simulink model "SF033A_VehSigCdng"  (R2013b)
settings: Solver=FixedStepDiscrete  StartTime=0.0  StopTime=6  FixedStep=.002  RelTol=1e-3
model workspace (MAT data in the model file):
  SLAMConfig_1_ATPP = [3707764736; 2; 1; 1; 1; 34]
values from neighbouring files (symbols this model uses):
  ARCHGLBPRM_180OVERPI_ULS_F32 = DataDict.Constant    [SF033A_VehSigCdng_DataDict.m]
  ARCHGLBPRM_2MILLISEC_SEC_F32 = DataDict.Constant    [SF033A_VehSigCdng_DataDict.m]
  AUNITCNVN_KPHPERSECPERMTRPERSECSQD_F32 = DataDict.Constant    [SF033A_VehSigCdng_DataDict.m]
  FLTINJ_VEHSIGCDNG_SERLCOMVEHLATA = DataDict.Constant    [SF033A_VehSigCdng_DataDict.m]
  FLTINJ_VEHSIGCDNG_SERLCOMVEHLGTA = DataDict.Constant    [SF033A_VehSigCdng_DataDict.m]
  FLTINJ_VEHSIGCDNG_SERLCOMVEHSPD = DataDict.Constant    [SF033A_VehSigCdng_DataDict.m]
  FLTINJ_VEHSIGCDNG_SERLCOMVEHYAWRATE = DataDict.Constant    [SF033A_VehSigCdng_DataDict.m]
  KPHCONVTOMTRPERSEC_MTRPERSECPERKPH_F32 = DataDict.Constant    [SF033A_VehSigCdng_DataDict.m]
  VehSigCdngDftLatA = DataDict.Calibration    [SF033A_VehSigCdng_DataDict.m]
  VehSigCdngDftLgtA = DataDict.Calibration    [SF033A_VehSigCdng_DataDict.m]
  VehSigCdngDftVehSpd = DataDict.Calibration    [SF033A_VehSigCdng_DataDict.m]
  VehSigCdngDftYawRate = DataDict.Calibration    [SF033A_VehSigCdng_DataDict.m]
  VehSigCdngLatADifThd = DataDict.Calibration    [SF033A_VehSigCdng_DataDict.m]
  VehSigCdngLatASlewRate = DataDict.Calibration    [SF033A_VehSigCdng_DataDict.m]
  VehSigCdngLtgADifThd = DataDict.Calibration    [SF033A_VehSigCdng_DataDict.m]
  VehSigCdngLtgASlewRate = DataDict.Calibration    [SF033A_VehSigCdng_DataDict.m]
  VehSigCdngVehSpdDifThd = DataDict.Calibration    [SF033A_VehSigCdng_DataDict.m]
  VehSigCdngVehSpdSlewRate = DataDict.Calibration    [SF033A_VehSigCdng_DataDict.m]
  VehSigCdngVehYawSlewRate = DataDict.Calibration    [SF033A_VehSigCdng_DataDict.m]
  VehSigCdngYawRateDifThd = DataDict.Calibration    [SF033A_VehSigCdng_DataDict.m]
  VEHSPDOVRDHWTQTHD_HWNWTMTR_F32 = DataDict.Constant    [SF033A_VehSigCdng_DataDict.m]
libraries: NxtrLim x9, Fil x4, simulink x1
(part 2 of 3)

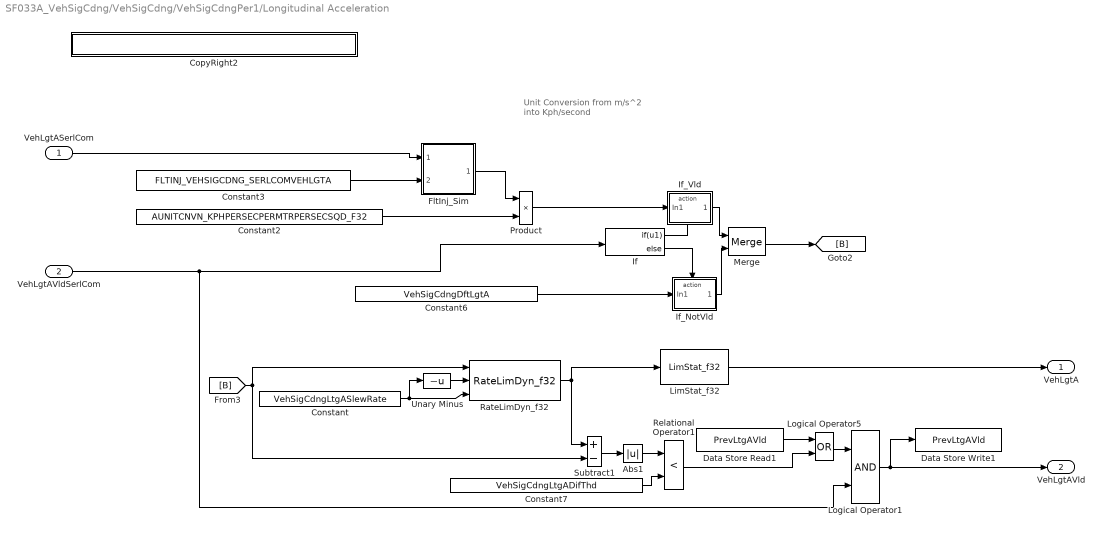
== system SF033A_VehSigCdng/VehSigCdng/VehSigCdngPer1/Longitudinal Acceleration ==
  note: Unit Conversion from
      | m/s^2 into Kph/second
  VehLgtASerlCom : Inport  RequirementInfo="{'linktype_rmi_doors' '00012fc2 (/E-STEER Core/SubSystem Specifications/Application Functions - EA4/SF033A Vehicle Signal Conditioning)' '#SF033A_86' 'true' 'REQ:  SF033A_86' '' ; 'linktype_rmi_doors' '00012fc2 (/E-STEER Core/SubSystem Specifications/Application Functions - EA4/SF033A Vehicle Signal Conditioning)' '#SF033A_82' 'true' 'REQ:  SF033A_82' '' } %GIDa_33bbc02e_3c9f_42eb_b3cb_1f1096c685a4"  PortDimensions=1
  VehLgtAVldSerlCom : Inport  RequirementInfo="{'linktype_rmi_doors' '00012fc2 (/E-STEER Core/SubSystem Specifications/Application Functions - EA4/SF033A Vehicle Signal Conditioning)' '#SF033A_86' 'true' 'REQ:  SF033A_86' '' ; 'linktype_rmi_doors' '00012fc2 (/E-STEER Core/SubSystem Specifications/Application Functions - EA4/SF033A Vehicle Signal Conditioning)' '#SF033A_82' 'true' 'REQ:  SF033A_82' '' } %GIDa_e6b17e37_5584_47ea_92c0_6fe41260cb29"  Port=2  PortDimensions=1
  Abs1 : Abs  RequirementInfo="{'linktype_rmi_doors' '00012fc2 (/E-STEER Core/SubSystem Specifications/Application Functions - EA4/SF033A Vehicle Signal Conditioning)' '#SF033A_84' 'true' 'REQ:  SF033A_84' '' } %GIDa_797c561b_561e_4e44_b4de_5fe8774172b8"
  Constant : Constant  RequirementInfo="{'linktype_rmi_doors' '00012fc2 (/E-STEER Core/SubSystem Specifications/Application Functions - EA4/SF033A Vehicle Signal Conditioning)' '#SF033A_85' 'true' 'REQ:  SF033A_85' '' } %GIDa_d723961e_7ba0_4e7b_8761_b2c80f0d3b1d"  Value=VehSigCdngLtgASlewRate
  Constant2 : Constant  RequirementInfo="{'linktype_rmi_doors' '00012fc2 (/E-STEER Core/SubSystem Specifications/Application Functions - EA4/SF033A Vehicle Signal Conditioning)' '#SF033A_59' 'true' 'REQ:  SF033A_59' '' } %GIDa_ec856914_362d_4179_a54b_12fbeb9435f3"  Value=AUNITCNVN_KPHPERSECPERMTRPERSECSQD_F32  VectorParams1D=off
      settings: AttributesFormatString=Interpret vector parameters as 1-D: %<VectorParams1D>
  Constant3 : Constant  RequirementInfo="{'linktype_rmi_doors' '00012fc2 (/E-STEER Core/SubSystem Specifications/Application Functions - EA4/SF033A Vehicle Signal Conditioning)' '#SF033A_108' 'true' 'REQ:  SF033A_108' '' } %GIDa_e621928c_ce46_4adf_8fc4_0ef521a724f5"  Value=FLTINJ_VEHSIGCDNG_SERLCOMVEHLGTA
  Constant6 : Constant  RequirementInfo="{'linktype_rmi_doors' '00012fc2 (/E-STEER Core/SubSystem Specifications/Application Functions - EA4/SF033A Vehicle Signal Conditioning)' '#SF033A_82' 'true' 'REQ:  SF033A_82' '' } %GIDa_38656e99_4cc9_4ca6_97fe_baf14fa5e910"  Value=VehSigCdngDftLgtA
  Constant7 : Constant  RequirementInfo="{'linktype_rmi_doors' '00012fc2 (/E-STEER Core/SubSystem Specifications/Application Functions - EA4/SF033A Vehicle Signal Conditioning)' '#SF033A_84' 'true' 'REQ:  SF033A_84' '' } %GIDa_a6bcb836_9e09_47f4_95b1_6135acfd8dce"  Value=VehSigCdngLtgADifThd
  CopyRight2 : Subsystem  Description=|  mask(Copyright Information){none=on}
      | Copyright info block.                                               
      |                                                                     
      | Place copyright information at the top of every subsystem in design.
      mask prompts: none "No parameters"
      mask help: Place copyright information at the top of every subsystem in design.
      mask Display:
      | NxtrConf = 'Nexteer Confidential';
      | 
      | sys = bdroot; %handle for the current model ("system")
      | first = get_param(sys,'Created');
      | first = first(end-3:end);  %year is last four digits
      | 
      | last = get_param(sys,'LastModifiedDate');
      | if isempty(last)
      |     last = datestr(now,'yyyy');
      | else
      |     last = last(end-3:end);
      | end
      | 
      | if strcmp(first,last)
      |     fprintf('%s -- Copyright %s Nexteer',NxtrConf,first)
      | else
      |     fprintf('%s -- %s%s- %s Nexteer',NxtrConf,char(169),first,last)
      | end
  Data Store Read1 : DataStoreRead  DataStoreName=PrevLtgAVld
  Data Store Write1 : DataStoreWrite  DataStoreName=PrevLtgAVld
  FltInj_Sim : Subsystem  RequirementInfo="{'linktype_rmi_doors' '00012fc2 (/E-STEER Core/SubSystem Specifications/Application Functions - EA4/SF033A Vehicle Signal Conditioning)' '#SF033A_108' 'true' 'REQ:  SF033A_108' '' } %GIDa_c93a5ef0_41d3_4b11_8d99_12e677f7689f"  TreatAsAtomicUnit=on  VariantControl=FltInj_sim
  If : If  RequirementInfo="{'linktype_rmi_doors' '00012fc2 (/E-STEER Core/SubSystem Specifications/Application Functions - EA4/SF033A Vehicle Signal Conditioning)' '#SF033A_86' 'true' 'REQ:  SF033A_86' '' } %GIDa_505aabb8_9ea7_4ce8_ab09_e77c025f66a2"  IfExpression=u1
  If_NotVld : Subsystem  RequirementInfo="{'linktype_rmi_doors' '00012fc2 (/E-STEER Core/SubSystem Specifications/Application Functions - EA4/SF033A Vehicle Signal Conditioning)' '#SF033A_82' 'true' 'REQ:  SF033A_82' '' } %GIDa_ee273562_eb50_4af6_ac31_a51d74597282"  TreatAsAtomicUnit=on
  If_Vld : Subsystem  RequirementInfo="{'linktype_rmi_doors' '00012fc2 (/E-STEER Core/SubSystem Specifications/Application Functions - EA4/SF033A Vehicle Signal Conditioning)' '#SF033A_86' 'true' 'REQ:  SF033A_86' '' } %GIDa_33575e89_f28b_438e_83bd_26ce1620f961"  TreatAsAtomicUnit=on
  LimStat_f32 : NxtrLim/LimStat_f32  RequirementInfo="{'linktype_rmi_doors' '00012fc2 (/E-STEER Core/SubSystem Specifications/Application Functions - EA4/SF033A Vehicle Signal Conditioning)' '#SF033A_68' 'true' 'REQ:  SF033A_68' '' } %GIDa_18436023_bcbe_4abf_86ab_3c62b00c008d"  LoLim=VEHLGTAMINLIM_KPHPERSEC_F32  HiLim=VEHLGTAMAXLIM_KPHPERSEC_F32
      settings: AttributesFormatString=|
      | Low Limit: %<LoLim>
      | High Limit:%<HiLim>
  Logical Operator1 : Logic  RequirementInfo="{'linktype_rmi_doors' '00012fc2 (/E-STEER Core/SubSystem Specifications/Application Functions - EA4/SF033A Vehicle Signal Conditioning)' '#SF033A_84' 'true' 'REQ:  SF033A_84' '' } %GIDa_91902d41_af99_47de_aab0_360b5ef293e4"  AllPortsSameDT=off  OutDataTypeStr=boolean
  Logical Operator5 : Logic  RequirementInfo={} %GIDa_8d4a0e43_fe65_49db_b57f_50a3f4f94ca0  Operator=OR  AllPortsSameDT=off  OutDataTypeStr=boolean
  Merge : Merge  RequirementInfo="{'linktype_rmi_doors' '00012fc2 (/E-STEER Core/SubSystem Specifications/Application Functions - EA4/SF033A Vehicle Signal Conditioning)' '#SF033A_86' 'true' 'REQ:  SF033A_86' '' ; 'linktype_rmi_doors' '00012fc2 (/E-STEER Core/SubSystem Specifications/Application Functions - EA4/SF033A Vehicle Signal Conditioning)' '#SF033A_82' 'true' 'REQ:  SF033A_82' '' } %GIDa_983fbb98_8f0c_4570_9d68_9c32efc81a5d"
  Product : Product  RequirementInfo="{'linktype_rmi_doors' '00012fc2 (/E-STEER Core/SubSystem Specifications/Application Functions - EA4/SF033A Vehicle Signal Conditioning)' '#SF033A_59' 'true' 'REQ:  SF033A_59' '' } %GIDa_1eeee2f6_c5ba_4cb6_9814_ba10eb593775"
  RateLimDyn_f32 : NxtrLim/RateLimDyn_f32  RequirementInfo="{'linktype_rmi_doors' '00012fc2 (/E-STEER Core/SubSystem Specifications/Application Functions - EA4/SF033A Vehicle Signal Conditioning)' '#SF033A_85' 'true' 'REQ:  SF033A_85' '' ; 'linktype_rmi_doors' '00012fc2 (/E-STEER Core/SubSystem Specifications/Application Functions - EA4/SF033A Vehicle Signal Conditioning)' '#SF033A_84' 'true' 'REQ:  SF033A_84' '' } %GIDa_0f96da6e_a085_4a67_b551_d12168310f23"  StVar=PrevLtgA  Ts=ARCHGLBPRM_2MILLISEC_SEC_F32
      settings: AttributesFormatString=StVar: %<StVar>
  Relational Operator1 : RelationalOperator  RequirementInfo="{'linktype_rmi_doors' '00012fc2 (/E-STEER Core/SubSystem Specifications/Application Functions - EA4/SF033A Vehicle Signal Conditioning)' '#SF033A_84' 'true' 'REQ:  SF033A_84' '' } %GIDa_82a5ab49_6f2e_40dc_b5a9_75231274a681"  Operator=<  OutDataTypeStr=boolean
  Subtract1 : Sum  RequirementInfo="{'linktype_rmi_doors' '00012fc2 (/E-STEER Core/SubSystem Specifications/Application Functions - EA4/SF033A Vehicle Signal Conditioning)' '#SF033A_84' 'true' 'REQ:  SF033A_84' '' } %GIDa_7318186c_1940_4faa_a34f_d2aceaf8209d"  Inputs=+-
  Unary Minus : UnaryMinus  RequirementInfo="{'linktype_rmi_doors' '00012fc2 (/E-STEER Core/SubSystem Specifications/Application Functions - EA4/SF033A Vehicle Signal Conditioning)' '#SF033A_85' 'true' 'REQ:  SF033A_85' '' } %GIDa_97d8531e_46c4_4ccd_8741_b4d188cb9804"
  VehLgtA : Outport  RequirementInfo="{'linktype_rmi_doors' '00012fc2 (/E-STEER Core/SubSystem Specifications/Application Functions - EA4/SF033A Vehicle Signal Conditioning)' '#SF033A_86' 'true' 'REQ:  SF033A_86' '' ; 'linktype_rmi_doors' '00012fc2 (/E-STEER Core/SubSystem Specifications/Application Functions - EA4/SF033A Vehicle Signal Conditioning)' '#SF033A_82' 'true' 'REQ:  SF033A_82' '' } %GIDa_61c91e13_416a_4925_b029_01b27432960c"  PortDimensions=1
  VehLgtAVld : Outport  RequirementInfo="{'linktype_rmi_doors' '00012fc2 (/E-STEER Core/SubSystem Specifications/Application Functions - EA4/SF033A Vehicle Signal Conditioning)' '#SF033A_86' 'true' 'REQ:  SF033A_86' '' ; 'linktype_rmi_doors' '00012fc2 (/E-STEER Core/SubSystem Specifications/Application Functions - EA4/SF033A Vehicle Signal Conditioning)' '#SF033A_82' 'true' 'REQ:  SF033A_82' '' } %GIDa_c1efd084_9a11_443e_acd8_34c2b5bdb0c0"  Port=2  PortDimensions=1
  wires:
  Constant2/1 -> Product/2
  Constant3/1 -> FltInj_Sim/2(Enum)
  Subtract1/1 -> Abs1/1
  Abs1/1 -> Relational Operator1/1
  Constant7/1 -> Relational Operator1/2
  [B] -> RateLimDyn_f32/1, Subtract1/2
  VehLgtAVldSerlCom/1 -> If/1, Logical Operator1/2
  LimStat_f32/1 -> VehLgtA/1
  RateLimDyn_f32/1 -> LimStat_f32/1, Subtract1/1
  VehLgtASerlCom/1 -> FltInj_Sim/1(Signal)
  FltInj_Sim/1(Out1) -> Product/1
  Data Store Read1/1 -> Logical Operator5/1
  Logical Operator5/1 -> Logical Operator1/1
  Logical Operator1/1 -> VehLgtAVld/1, Data Store Write1/1
  Relational Operator1/1 -> Logical Operator5/2
  If/1 -> If_Vld/Action
  If/2 -> If_NotVld/Action
  If_Vld/1(Out1) -> Merge/1
  If_NotVld/1(Out1) -> Merge/2
  Constant6/1 -> If_NotVld/1(In1)
  Product/1 -> If_Vld/1(In1)
  Merge/1 -> [B]
  Unary Minus/1 -> RateLimDyn_f32/2
  Constant/1 -> RateLimDyn_f32/3, Unary Minus/1

== stateflow chart SF033A_VehSigCdng/Chart ==
  state Trigger
    on every(1,event): per1;
  (default) -> Trigger : {
      | per;
      | }
  events: event input FUNCTION_CALL_EVENT; per output FUNCTION_CALL_EVENT; per1 output FUNCTION_CALL_EVENT

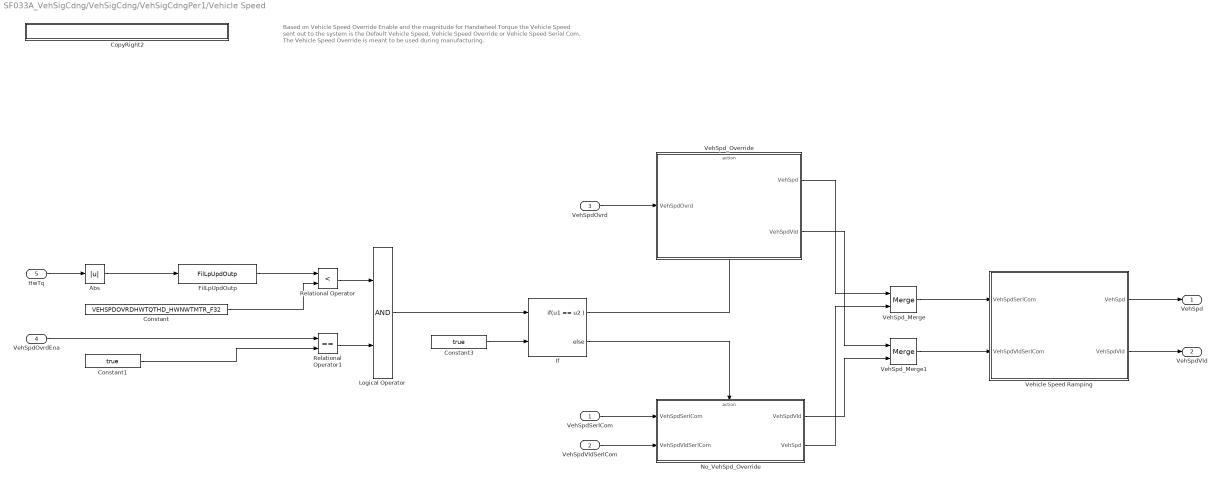
== system SF033A_VehSigCdng/VehSigCdng/VehSigCdngPer1/Vehicle Speed ==
  note: Based on Vehicle Speed Override Enable and the magnitude for Handwheel Torque the Vehicle Speed
      | sent out to the system is the Default Vehicle Speed, Vehicle Speed Override or Vehicle Speed Serial Com.
      |
      | The Vehicle Speed Override is meant to be used during manufacturing.
  VehSpdSerlCom : Inport  RequirementInfo="{'linktype_rmi_doors' '00012fc2 (/E-STEER Core/SubSystem Specifications/Application Functions - EA4/SF033A Vehicle Signal Conditioning)' '#SF033A_83' 'true' 'REQ:  SF033A_83' '' ; 'linktype_rmi_doors' '00012fc2 (/E-STEER Core/SubSystem Specifications/Application Functions - EA4/SF033A Vehicle Signal Conditioning)' '#SF033A_75' 'true' 'REQ:  SF033A_75' '' } %GIDa_50e47d90_d3f5_4aae_a8e9_451591674adf"  PortDimensions=1
  VehSpdVldSerlCom : Inport  RequirementInfo="{'linktype_rmi_doors' '00012fc2 (/E-STEER Core/SubSystem Specifications/Application Functions - EA4/SF033A Vehicle Signal Conditioning)' '#SF033A_83' 'true' 'REQ:  SF033A_83' '' ; 'linktype_rmi_doors' '00012fc2 (/E-STEER Core/SubSystem Specifications/Application Functions - EA4/SF033A Vehicle Signal Conditioning)' '#SF033A_75' 'true' 'REQ:  SF033A_75' '' } %GIDa_49df1e48_5853_4226_9564_056e90acf9b5"  Port=2  PortDimensions=1
  VehSpdOvrd : Inport  RequirementInfo="{'linktype_rmi_doors' '00012fc2 (/E-STEER Core/SubSystem Specifications/Application Functions - EA4/SF033A Vehicle Signal Conditioning)' '#SF033A_70' 'true' 'REQ:  SF033A_70' '' ; 'linktype_rmi_doors' '00012fc2 (/E-STEER Core/SubSystem Specifications/Application Functions - EA4/SF033A Vehicle Signal Conditioning)' '#SF033A_106' 'true' 'REQ:  SF033A_106' '' } %GIDa_d49c07b2_9621_4ad6_936a_0a97cd6ed3de"  Port=3  PortDimensions=1
  VehSpdOvrdEna : Inport  RequirementInfo="{'linktype_rmi_doors' '00012fc2 (/E-STEER Core/SubSystem Specifications/Application Functions - EA4/SF033A Vehicle Signal Conditioning)' '#SF033A_70' 'true' 'REQ:  SF033A_70' '' ; 'linktype_rmi_doors' '00012fc2 (/E-STEER Core/SubSystem Specifications/Application Functions - EA4/SF033A Vehicle Signal Conditioning)' '#SF033A_106' 'true' 'REQ:  SF033A_106' '' } %GIDa_55540332_36a6_4d4c_9cf8_f0ef12908b37"  Port=4  PortDimensions=1
  HwTq : Inport  RequirementInfo="{'linktype_rmi_doors' '00012fc2 (/E-STEER Core/SubSystem Specifications/Application Functions - EA4/SF033A Vehicle Signal Conditioning)' '#SF033A_70' 'true' 'REQ:  SF033A_70' '' ; 'linktype_rmi_doors' '00012fc2 (/E-STEER Core/SubSystem Specifications/Application Functions - EA4/SF033A Vehicle Signal Conditioning)' '#SF033A_106' 'true' 'REQ:  SF033A_106' '' } %GIDa_d2e07287_5722_4a7d_ba43_cea7066e677d"  Port=5  PortDimensions=1
  Abs : Abs  RequirementInfo="{'linktype_rmi_doors' '00012fc2 (/E-STEER Core/SubSystem Specifications/Application Functions - EA4/SF033A Vehicle Signal Conditioning)' '#SF033A_70' 'true' 'REQ:  SF033A_70' '' ; 'linktype_rmi_doors' '00012fc2 (/E-STEER Core/SubSystem Specifications/Application Functions - EA4/SF033A Vehicle Signal Conditioning)' '#SF033A_106' 'true' 'REQ:  SF033A_106' '' } %GIDa_c208f1a3_0d63_48d9_aa05_42c2b808d7f0"
  Constant : Constant  RequirementInfo="{'linktype_rmi_doors' '00012fc2 (/E-STEER Core/SubSystem Specifications/Application Functions - EA4/SF033A Vehicle Signal Conditioning)' '#SF033A_70' 'true' 'REQ:  SF033A_70' '' ; 'linktype_rmi_doors' '00012fc2 (/E-STEER Core/SubSystem Specifications/Application Functions - EA4/SF033A Vehicle Signal Conditioning)' '#SF033A_106' 'true' 'REQ:  SF033A_106' '' } %GIDa_5e91e17d_823b_4957_86ab_bbbc595eb504"  Value=VEHSPDOVRDHWTQTHD_HWNWTMTR_F32
  Constant1 : Constant  RequirementInfo="{'linktype_rmi_doors' '00012fc2 (/E-STEER Core/SubSystem Specifications/Application Functions - EA4/SF033A Vehicle Signal Conditioning)' '#SF033A_70' 'true' 'REQ:  SF033A_70' '' ; 'linktype_rmi_doors' '00012fc2 (/E-STEER Core/SubSystem Specifications/Application Functions - EA4/SF033A Vehicle Signal Conditioning)' '#SF033A_106' 'true' 'REQ:  SF033A_106' '' } %GIDa_a2d5b041_1199_45d3_be7c_a18290b1e2ee"  Value=true
  Constant3 : Constant  RequirementInfo="{'linktype_rmi_doors' '00012fc2 (/E-STEER Core/SubSystem Specifications/Application Functions - EA4/SF033A Vehicle Signal Conditioning)' '#SF033A_70' 'true' 'REQ:  SF033A_70' '' ; 'linktype_rmi_doors' '00012fc2 (/E-STEER Core/SubSystem Specifications/Application Functions - EA4/SF033A Vehicle Signal Conditioning)' '#SF033A_106' 'true' 'REQ:  SF033A_106' '' } %GIDa_ad796ebb_5a8e_4eb1_9daa_b89bf1516966"  Value=true
  CopyRight2 : Subsystem  Description=|  mask(Copyright Information){none=on}
      | Copyright info block.                                               
      |                                                                     
      | Place copyright information at the top of every subsystem in design.
      mask prompts: none "No parameters"
      mask help: Place copyright information at the top of every subsystem in design.
      mask Display:
      | NxtrConf = 'Nexteer Confidential';
      | 
      | sys = bdroot; %handle for the current model ("system")
      | first = get_param(sys,'Created');
      | first = first(end-3:end);  %year is last four digits
      | 
      | last = get_param(sys,'LastModifiedDate');
      | if isempty(last)
      |     last = datestr(now,'yyyy');
      | else
      |     last = last(end-3:end);
      | end
      | 
      | if strcmp(first,last)
      |     fprintf('%s -- Copyright %s Nexteer',NxtrConf,first)
      | else
      |     fprintf('%s -- %s%s- %s Nexteer',NxtrConf,char(169),first,last)
      | end
  FilLpUpdOutp : Fil/FilLpUpdOutp  RequirementInfo="{'linktype_rmi_doors' '00012fc2 (/E-STEER Core/SubSystem Specifications/Application Functions - EA4/SF033A Vehicle Signal Conditioning)' '#SF033A_70' 'true' 'REQ:  SF033A_70' '' ; 'linktype_rmi_doors' '00012fc2 (/E-STEER Core/SubSystem Specifications/Application Functions - EA4/SF033A Vehicle Signal Conditioning)' '#SF033A_106' 'true' 'REQ:  SF033A_106' '' } %GIDa_f79bc1cc_33b0_4169_bb7f_beebdf37309b"  StVar=HwTqFilRec
      settings: AttributesFormatString=StVar: %<StVar>
  If : If  RequirementInfo="{'linktype_rmi_doors' '00012fc2 (/E-STEER Core/SubSystem Specifications/Application Functions - EA4/SF033A Vehicle Signal Conditioning)' '#SF033A_70' 'true' 'REQ:  SF033A_70' '' ; 'linktype_rmi_doors' '00012fc2 (/E-STEER Core/SubSystem Specifications/Application Functions - EA4/SF033A Vehicle Signal Conditioning)' '#SF033A_106' 'true' 'REQ:  SF033A_106' '' } %GIDa_6a17ea79_fa1c_4b98_8c4e_5d6af19a7612"  NumInputs=2  IfExpression=u1 == u2
  Logical Operator : Logic  RequirementInfo="{'linktype_rmi_doors' '00012fc2 (/E-STEER Core/SubSystem Specifications/Application Functions - EA4/SF033A Vehicle Signal Conditioning)' '#SF033A_70' 'true' 'REQ:  SF033A_70' '' ; 'linktype_rmi_doors' '00012fc2 (/E-STEER Core/SubSystem Specifications/Application Functions - EA4/SF033A Vehicle Signal Conditioning)' '#SF033A_106' 'true' 'REQ:  SF033A_106' '' } %GIDa_60bc963b_b4ae_406f_aa7c_41745d4504ac"  AllPortsSameDT=off  OutDataTypeStr=boolean
  No_VehSpd_Override : Subsystem  RequirementInfo="{'linktype_rmi_doors' '00012fc2 (/E-STEER Core/SubSystem Specifications/Application Functions - EA4/SF033A Vehicle Signal Conditioning)' '#SF033A_83' 'true' 'REQ:  SF033A_83' '' ; 'linktype_rmi_doors' '00012fc2 (/E-STEER Core/SubSystem Specifications/Application Functions - EA4/SF033A Vehicle Signal Conditioning)' '#SF033A_75' 'true' 'REQ:  SF033A_75' '' } %GIDa_e9b7843b_c4fc_41b0_bb01_4032fd5c080b"  TreatAsAtomicUnit=on
  Relational Operator : RelationalOperator  RequirementInfo="{'linktype_rmi_doors' '00012fc2 (/E-STEER Core/SubSystem Specifications/Application Functions - EA4/SF033A Vehicle Signal Conditioning)' '#SF033A_70' 'true' 'REQ:  SF033A_70' '' ; 'linktype_rmi_doors' '00012fc2 (/E-STEER Core/SubSystem Specifications/Application Functions - EA4/SF033A Vehicle Signal Conditioning)' '#SF033A_106' 'true' 'REQ:  SF033A_106' '' } %GIDa_aa10390b_dedd_4f68_9332_f93643322ca9"  Operator=<  OutDataTypeStr=boolean
  Relational Operator1 : RelationalOperator  RequirementInfo="{'linktype_rmi_doors' '00012fc2 (/E-STEER Core/SubSystem Specifications/Application Functions - EA4/SF033A Vehicle Signal Conditioning)' '#SF033A_70' 'true' 'REQ:  SF033A_70' '' ; 'linktype_rmi_doors' '00012fc2 (/E-STEER Core/SubSystem Specifications/Application Functions - EA4/SF033A Vehicle Signal Conditioning)' '#SF033A_106' 'true' 'REQ:  SF033A_106' '' } %GIDa_be71f559_dc97_42cb_8ec8_4564ed121948"  Operator===  OutDataTypeStr=boolean
  VehSpd_Merge : Merge
  VehSpd_Merge1 : Merge
  VehSpd_Override : Subsystem  RequirementInfo="{'linktype_rmi_doors' '00012fc2 (/E-STEER Core/SubSystem Specifications/Application Functions - EA4/SF033A Vehicle Signal Conditioning)' '#SF033A_70' 'true' 'REQ:  SF033A_70' '' ; 'linktype_rmi_doors' '00012fc2 (/E-STEER Core/SubSystem Specifications/Application Functions - EA4/SF033A Vehicle Signal Conditioning)' '#SF033A_106' 'true' 'REQ:  SF033A_106' '' } %GIDa_64635b2f_5587_48f5_a908_b376eb97f6fc"  TreatAsAtomicUnit=on
  Vehicle Speed Ramping : Subsystem  RequirementInfo="{'linktype_rmi_doors' '00012fc2 (/E-STEER Core/SubSystem Specifications/Application Functions - EA4/SF033A Vehicle Signal Conditioning)' '#SF033A_76' 'true' 'REQ:  SF033A_76' '' ; 'linktype_rmi_doors' '00012fc2 (/E-STEER Core/SubSystem Specifications/Application Functions - EA4/SF033A Vehicle Signal Conditioning)' '#SF033A_77' 'true' 'REQ:  SF033A_77' '' ; 'linktype_rmi_doors' '00012fc2 (/E-STEER Core/SubSystem Specifications/Application Functions - EA4/SF033A Vehicle Signal Conditioning)' '#SF033A_83' 'true' 'REQ:  SF033A_83' '' ; 'linktype_rmi_doors' '00012fc2 (/E-STEER Core/SubSystem Specifications/Application Functions - EA4/SF033A Vehicle Signal Conditioning)' '#SF033A_75' 'true' 'REQ:  SF033A_75' '' } %GIDa_12595cd6_985e_4719_99f0_1e7b173c1c54"
  VehSpd : Outport  RequirementInfo="{'linktype_rmi_doors' '00012fc2 (/E-STEER Core/SubSystem Specifications/Application Functions - EA4/SF033A Vehicle Signal Conditioning)' '#SF033A_83' 'true' 'REQ:  SF033A_83' '' ; 'linktype_rmi_doors' '00012fc2 (/E-STEER Core/SubSystem Specifications/Application Functions - EA4/SF033A Vehicle Signal Conditioning)' '#SF033A_75' 'true' 'REQ:  SF033A_75' '' } %GIDa_1b45b11b_fa1f_4891_8431_e23ac9934e1e"  PortDimensions=1
  VehSpdVld : Outport  RequirementInfo="{'linktype_rmi_doors' '00012fc2 (/E-STEER Core/SubSystem Specifications/Application Functions - EA4/SF033A Vehicle Signal Conditioning)' '#SF033A_83' 'true' 'REQ:  SF033A_83' '' ; 'linktype_rmi_doors' '00012fc2 (/E-STEER Core/SubSystem Specifications/Application Functions - EA4/SF033A Vehicle Signal Conditioning)' '#SF033A_75' 'true' 'REQ:  SF033A_75' '' } %GIDa_582d93a4_364b_4cf2_a56b_cc64ace1f74e"  Port=2  PortDimensions=1
  wires:
  VehSpd_Merge/1 -> Vehicle Speed Ramping/1(VehSpdSerlCom)
  Logical Operator/1 -> If/1
  Constant3/1 -> If/2
  If/1 -> VehSpd_Override/Action
  If/2 -> No_VehSpd_Override/Action
  VehSpdOvrd/1 -> VehSpd_Override/1(VehSpdOvrd)
  VehSpd_Override/1(VehSpd) -> VehSpd_Merge/1
  No_VehSpd_Override/2(VehSpd) -> VehSpd_Merge/2
  VehSpdSerlCom/1 -> No_VehSpd_Override/1(VehSpdSerlCom)
  VehSpdVldSerlCom/1 -> No_VehSpd_Override/2(VehSpdVldSerlCom)
  VehSpd_Merge1/1 -> Vehicle Speed Ramping/2(VehSpdVldSerlCom)
  Vehicle Speed Ramping/2(VehSpdVld) -> VehSpdVld/1
  Vehicle Speed Ramping/1(VehSpd) -> VehSpd/1
  VehSpdOvrdEna/1 -> Relational Operator1/1
  Constant1/1 -> Relational Operator1/2
  Constant/1 -> Relational Operator/2
  Relational Operator/1 -> Logical Operator/1
  Relational Operator1/1 -> Logical Operator/2
  VehSpd_Override/2(VehSpdVld) -> VehSpd_Merge1/1
  No_VehSpd_Override/1(VehSpdVld) -> VehSpd_Merge1/2
  HwTq/1 -> Abs/1
  Abs/1 -> FilLpUpdOutp/1
  FilLpUpdOutp/1 -> Relational Operator/1

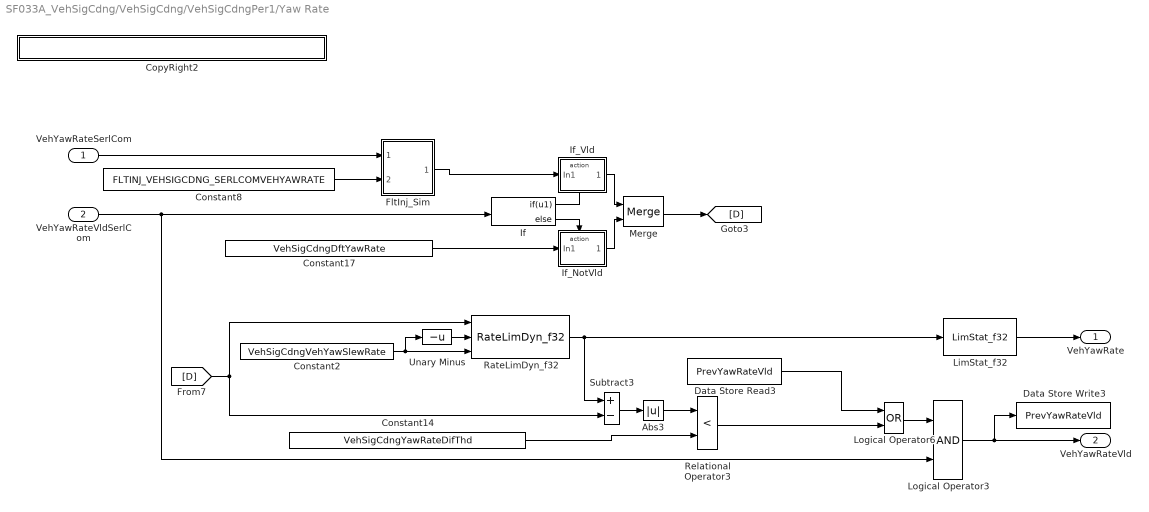
== system SF033A_VehSigCdng/VehSigCdng/VehSigCdngPer1/Yaw Rate  ==
  VehYawRateSerlCom : Inport  RequirementInfo="{'linktype_rmi_doors' '00012fc2 (/E-STEER Core/SubSystem Specifications/Application Functions - EA4/SF033A Vehicle Signal Conditioning)' '#SF033A_103' 'true' 'REQ:  SF033A_103' '' ; 'linktype_rmi_doors' '00012fc2 (/E-STEER Core/SubSystem Specifications/Application Functions - EA4/SF033A Vehicle Signal Conditioning)' '#SF033A_104' 'true' 'REQ:  SF033A_104' '' } %GIDa_42327bab_1a42_44b0_aac6_bf57499f9d4a"  PortDimensions=1
  VehYawRateVldSerlCom : Inport  RequirementInfo="{'linktype_rmi_doors' '00012fc2 (/E-STEER Core/SubSystem Specifications/Application Functions - EA4/SF033A Vehicle Signal Conditioning)' '#SF033A_103' 'true' 'REQ:  SF033A_103' '' ; 'linktype_rmi_doors' '00012fc2 (/E-STEER Core/SubSystem Specifications/Application Functions - EA4/SF033A Vehicle Signal Conditioning)' '#SF033A_104' 'true' 'REQ:  SF033A_104' '' } %GIDa_7753a280_7d89_4348_885e_6034bf751924"  Port=2  PortDimensions=1
  Abs3 : Abs  RequirementInfo="{'linktype_rmi_doors' '00012fc2 (/E-STEER Core/SubSystem Specifications/Application Functions - EA4/SF033A Vehicle Signal Conditioning)' '#SF033A_102' 'true' 'REQ:  SF033A_102' '' } %GIDa_4fb32f4a_392d_460c_ba61_5bad7a7fe4e0"
  Constant14 : Constant  RequirementInfo="{'linktype_rmi_doors' '00012fc2 (/E-STEER Core/SubSystem Specifications/Application Functions - EA4/SF033A Vehicle Signal Conditioning)' '#SF033A_102' 'true' 'REQ:  SF033A_102' '' } %GIDa_da74054d_82fc_49d9_a856_e4a728541d39"  Value=VehSigCdngYawRateDifThd
  Constant17 : Constant  RequirementInfo="{'linktype_rmi_doors' '00012fc2 (/E-STEER Core/SubSystem Specifications/Application Functions - EA4/SF033A Vehicle Signal Conditioning)' '#SF033A_104' 'true' 'REQ:  SF033A_104' '' } %GIDa_dd1b79a1_2d36_4bc4_96ce_1f418b544af1"  Value=VehSigCdngDftYawRate
  Constant2 : Constant  RequirementInfo="{'linktype_rmi_doors' '00012fc2 (/E-STEER Core/SubSystem Specifications/Application Functions - EA4/SF033A Vehicle Signal Conditioning)' '#SF033A_101' 'true' 'REQ:  SF033A_101' '' } %GIDa_0b8d7c78_70af_46f4_bdb6_22bde9c55af9"  Value=VehSigCdngVehYawSlewRate
  Constant8 : Constant  RequirementInfo="{'linktype_rmi_doors' '00012fc2 (/E-STEER Core/SubSystem Specifications/Application Functions - EA4/SF033A Vehicle Signal Conditioning)' '#SF033A_110' 'true' 'REQ:  SF033A_110' '' } %GIDa_2ef17570_487b_420a_b242_60e3641662d0"  Value=FLTINJ_VEHSIGCDNG_SERLCOMVEHYAWRATE
  CopyRight2 : Subsystem  Description=|  mask(Copyright Information){none=on}
      | Copyright info block.                                               
      |                                                                     
      | Place copyright information at the top of every subsystem in design.
      mask prompts: none "No parameters"
      mask help: Place copyright information at the top of every subsystem in design.
      mask Display:
      | NxtrConf = 'Nexteer Confidential';
      | 
      | sys = bdroot; %handle for the current model ("system")
      | first = get_param(sys,'Created');
      | first = first(end-3:end);  %year is last four digits
      | 
      | last = get_param(sys,'LastModifiedDate');
      | if isempty(last)
      |     last = datestr(now,'yyyy');
      | else
      |     last = last(end-3:end);
      | end
      | 
      | if strcmp(first,last)
      |     fprintf('%s -- Copyright %s Nexteer',NxtrConf,first)
      | else
      |     fprintf('%s -- %s%s- %s Nexteer',NxtrConf,char(169),first,last)
      | end
  Data Store Read3 : DataStoreRead  DataStoreName=PrevYawRateVld
  Data Store Write3 : DataStoreWrite  DataStoreName=PrevYawRateVld
  FltInj_Sim : Subsystem  RequirementInfo="{'linktype_rmi_doors' '00012fc2 (/E-STEER Core/SubSystem Specifications/Application Functions - EA4/SF033A Vehicle Signal Conditioning)' '#SF033A_110' 'true' 'REQ:  SF033A_110' '' } %GIDa_c1923de8_ac61_4992_a7a1_e3187713f203"  TreatAsAtomicUnit=on  VariantControl=FltInj_sim
  If : If  RequirementInfo="{'linktype_rmi_doors' '00012fc2 (/E-STEER Core/SubSystem Specifications/Application Functions - EA4/SF033A Vehicle Signal Conditioning)' '#SF033A_103' 'true' 'REQ:  SF033A_103' '' ; 'linktype_rmi_doors' '00012fc2 (/E-STEER Core/SubSystem Specifications/Application Functions - EA4/SF033A Vehicle Signal Conditioning)' '#SF033A_104' 'true' 'REQ:  SF033A_104' '' } %GIDa_c356b67a_9e37_4af4_ab85_f4a1cda7f81d"  IfExpression=u1
  If_NotVld : Subsystem  RequirementInfo="{'linktype_rmi_doors' '00012fc2 (/E-STEER Core/SubSystem Specifications/Application Functions - EA4/SF033A Vehicle Signal Conditioning)' '#SF033A_104' 'true' 'REQ:  SF033A_104' '' } %GIDa_14ae8dc8_3459_4d65_960c_c640d414dfe3"  TreatAsAtomicUnit=on
  If_Vld : Subsystem  RequirementInfo="{'linktype_rmi_doors' '00012fc2 (/E-STEER Core/SubSystem Specifications/Application Functions - EA4/SF033A Vehicle Signal Conditioning)' '#SF033A_103' 'true' 'REQ:  SF033A_103' '' } %GIDa_010ce6cb_18ef_4752_8d5d_916f4b5ad013"  TreatAsAtomicUnit=on
  LimStat_f32 : NxtrLim/LimStat_f32  RequirementInfo="{'linktype_rmi_doors' '00012fc2 (/E-STEER Core/SubSystem Specifications/Application Functions - EA4/SF033A Vehicle Signal Conditioning)' '#SF033A_68' 'true' 'REQ:  SF033A_68' '' } %GIDa_28146c31_06a3_4537_996d_464529f8f432"  LoLim=VEHYAWRATEMINLIM_VEHDEGPERSEC_F32  HiLim=VEHYAWRATEMAXLIM_VEHDEGPERSEC_F32
      settings: AttributesFormatString=|
      | Low Limit: %<LoLim>
      | High Limit:%<HiLim>
  Logical Operator3 : Logic  RequirementInfo="{'linktype_rmi_doors' '00012fc2 (/E-STEER Core/SubSystem Specifications/Application Functions - EA4/SF033A Vehicle Signal Conditioning)' '#SF033A_102' 'true' 'REQ:  SF033A_102' '' } %GIDa_08c21ea3_2b53_410e_b039_c617cb61884a"  AllPortsSameDT=off  OutDataTypeStr=boolean
  Logical Operator6 : Logic  RequirementInfo={} %GIDa_81e75219_2fd5_471c_8746_2bed17654001  Operator=OR  AllPortsSameDT=off  OutDataTypeStr=boolean
  Merge : Merge  RequirementInfo="{'linktype_rmi_doors' '00012fc2 (/E-STEER Core/SubSystem Specifications/Application Functions - EA4/SF033A Vehicle Signal Conditioning)' '#SF033A_103' 'true' 'REQ:  SF033A_103' '' ; 'linktype_rmi_doors' '00012fc2 (/E-STEER Core/SubSystem Specifications/Application Functions - EA4/SF033A Vehicle Signal Conditioning)' '#SF033A_104' 'true' 'REQ:  SF033A_104' '' } %GIDa_0c7a7cc4_ebec_4cdc_bfa1_44dfac9eecc7"
  RateLimDyn_f32 : NxtrLim/RateLimDyn_f32  RequirementInfo="{'linktype_rmi_doors' '00012fc2 (/E-STEER Core/SubSystem Specifications/Application Functions - EA4/SF033A Vehicle Signal Conditioning)' '#SF033A_101' 'true' 'REQ:  SF033A_101' '' } %GIDa_ab096e3e_ca22_49ea_9a63_a4bae17323ef"  StVar=PrevYawRate  Ts=ARCHGLBPRM_2MILLISEC_SEC_F32
      settings: AttributesFormatString=StVar: %<StVar>
  Relational Operator3 : RelationalOperator  RequirementInfo="{'linktype_rmi_doors' '00012fc2 (/E-STEER Core/SubSystem Specifications/Application Functions - EA4/SF033A Vehicle Signal Conditioning)' '#SF033A_102' 'true' 'REQ:  SF033A_102' '' } %GIDa_54f1ee31_9d4d_49fe_bc29_1748faf526b6"  Operator=<  OutDataTypeStr=boolean
  Subtract3 : Sum  RequirementInfo="{'linktype_rmi_doors' '00012fc2 (/E-STEER Core/SubSystem Specifications/Application Functions - EA4/SF033A Vehicle Signal Conditioning)' '#SF033A_102' 'true' 'REQ:  SF033A_102' '' } %GIDa_8e018a10_91c1_4140_b7f7_11674384166e"  Inputs=+-
  Unary Minus : UnaryMinus  RequirementInfo="{'linktype_rmi_doors' '00012fc2 (/E-STEER Core/SubSystem Specifications/Application Functions - EA4/SF033A Vehicle Signal Conditioning)' '#SF033A_101' 'true' 'REQ:  SF033A_101' '' } %GIDa_06b108ae_c05a_488f_8543_b97e1c2abca3"
  VehYawRate : Outport  RequirementInfo="{'linktype_rmi_doors' '00012fc2 (/E-STEER Core/SubSystem Specifications/Application Functions - EA4/SF033A Vehicle Signal Conditioning)' '#SF033A_103' 'true' 'REQ:  SF033A_103' '' ; 'linktype_rmi_doors' '00012fc2 (/E-STEER Core/SubSystem Specifications/Application Functions - EA4/SF033A Vehicle Signal Conditioning)' '#SF033A_104' 'true' 'REQ:  SF033A_104' '' } %GIDa_bc8c9bc7_dd7e_4385_a98d_5c352efa762b"  PortDimensions=1
  VehYawRateVld : Outport  RequirementInfo="{'linktype_rmi_doors' '00012fc2 (/E-STEER Core/SubSystem Specifications/Application Functions - EA4/SF033A Vehicle Signal Conditioning)' '#SF033A_103' 'true' 'REQ:  SF033A_103' '' ; 'linktype_rmi_doors' '00012fc2 (/E-STEER Core/SubSystem Specifications/Application Functions - EA4/SF033A Vehicle Signal Conditioning)' '#SF033A_104' 'true' 'REQ:  SF033A_104' '' } %GIDa_4d5b5c03_b8de_486e_a54e_9a7b8518c64d"  Port=2  PortDimensions=1
  wires:
  Subtract3/1 -> Abs3/1
  Abs3/1 -> Relational Operator3/1
  Constant14/1 -> Relational Operator3/2
  VehYawRateSerlCom/1 -> FltInj_Sim/1(Signal)
  Constant8/1 -> FltInj_Sim/2(Enum)
  RateLimDyn_f32/1 -> LimStat_f32/1, Subtract3/1
  LimStat_f32/1 -> VehYawRate/1
  VehYawRateVldSerlCom/1 -> Logical Operator3/2, If/1
  Logical Operator3/1 -> VehYawRateVld/1, Data Store Write3/1
  Relational Operator3/1 -> Logical Operator6/2
  Data Store Read3/1 -> Logical Operator6/1
  Logical Operator6/1 -> Logical Operator3/1
  If/1 -> If_Vld/Action
  If/2 -> If_NotVld/Action
  If_Vld/1(Out1) -> Merge/1
  If_NotVld/1(Out1) -> Merge/2
  Merge/1 -> [D]
  FltInj_Sim/1(Out1) -> If_Vld/1(In1)
  Constant17/1 -> If_NotVld/1(In1)
  [D] -> Subtract3/2, RateLimDyn_f32/1
  Constant2/1 -> RateLimDyn_f32/3, Unary Minus/1
  Unary Minus/1 -> RateLimDyn_f32/2

== system SF033A_VehSigCdng/VehSigCdng/VehSigCdngPer1/Lateral Acceleration/CopyRight2 ==

== system SF033A_VehSigCdng/VehSigCdng/VehSigCdngPer1/Lateral Acceleration/FltInj_Sim ==
  note: This block requires no modification by FDD author.
      |
      | This block does not actually simulate any fault injection.  It is simply a pass-thru.
      |
      | The Enum port (#2) simply terminates its signal, but we are trying to force the FDD author
      | to properly use the FltInjectionLocType enumeration in FDD model.
  note: EA4.x Fault Injection
  note: Inport #2 must be enumeration
      | Enum: FltInjectionLocType
  Signal : Inport
  Enum : Inport  Port=2
  Terminator : Terminator
  Out1 : Outport
  wires:
  Signal/1 -> Out1/1
  Enum/1 -> Terminator/1

== system SF033A_VehSigCdng/VehSigCdng/VehSigCdngPer1/Lateral Acceleration/If_Vld ==
  In1 : Inport
  Action Port : ActionPort  ActionType=then
  CopyRight2 : Subsystem  Description=|  mask(Copyright Information){none=on}
      | Copyright info block.                                               
      |                                                                     
      | Place copyright information at the top of every subsystem in design.
      mask prompts: none "No parameters"
      mask help: Place copyright information at the top of every subsystem in design.
      mask Display:
      | NxtrConf = 'Nexteer Confidential';
      | 
      | sys = bdroot; %handle for the current model ("system")
      | first = get_param(sys,'Created');
      | first = first(end-3:end);  %year is last four digits
      | 
      | last = get_param(sys,'LastModifiedDate');
      | if isempty(last)
      |     last = datestr(now,'yyyy');
      | else
      |     last = last(end-3:end);
      | end
      | 
      | if strcmp(first,last)
      |     fprintf('%s -- Copyright %s Nexteer',NxtrConf,first)
      | else
      |     fprintf('%s -- %s%s- %s Nexteer',NxtrConf,char(169),first,last)
      | end
  Out1 : Outport
  wires:
  In1/1 -> Out1/1

== system SF033A_VehSigCdng/VehSigCdng/VehSigCdngPer1/Lateral Acceleration/if_NotVld ==
  In1 : Inport
  Action Port : ActionPort  ActionType=else
  CopyRight2 : Subsystem  Description=|  mask(Copyright Information){none=on}
      | Copyright info block.                                               
      |                                                                     
      | Place copyright information at the top of every subsystem in design.
      mask prompts: none "No parameters"
      mask help: Place copyright information at the top of every subsystem in design.
      mask Display:
      | NxtrConf = 'Nexteer Confidential';
      | 
      | sys = bdroot; %handle for the current model ("system")
      | first = get_param(sys,'Created');
      | first = first(end-3:end);  %year is last four digits
      | 
      | last = get_param(sys,'LastModifiedDate');
      | if isempty(last)
      |     last = datestr(now,'yyyy');
      | else
      |     last = last(end-3:end);
      | end
      | 
      | if strcmp(first,last)
      |     fprintf('%s -- Copyright %s Nexteer',NxtrConf,first)
      | else
      |     fprintf('%s -- %s%s- %s Nexteer',NxtrConf,char(169),first,last)
      | end
  Out1 : Outport
  wires:
  In1/1 -> Out1/1

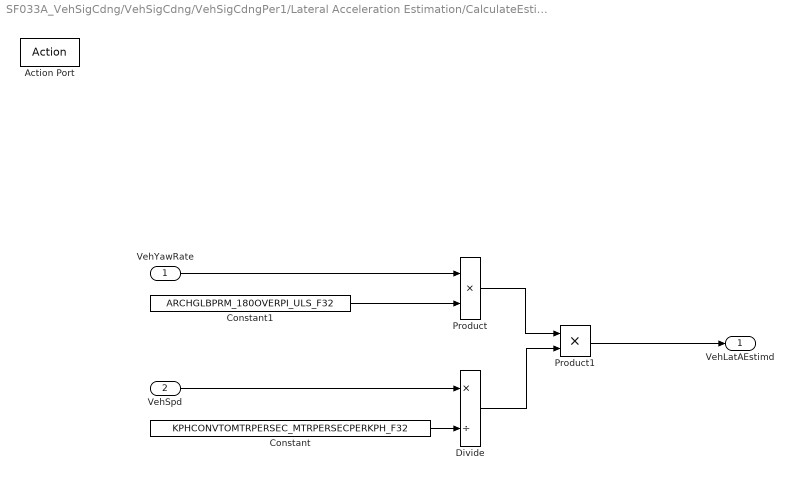
== system SF033A_VehSigCdng/VehSigCdng/VehSigCdngPer1/Lateral Acceleration Estimation/CalculateEstimate ==
  VehYawRate : Inport  RequirementInfo="{'linktype_rmi_doors' '00012fc2 (/E-STEER Core/SubSystem Specifications/Application Functions - EA4/SF033A Vehicle Signal Conditioning)' '#SF033A_97' 'true' 'REQ:  SF033A_97' '' } %GIDa_ff045a5f_e541_417a_86b2_5a23ac9bccc5"  PortDimensions=1
  VehSpd : Inport  RequirementInfo="{'linktype_rmi_doors' '00012fc2 (/E-STEER Core/SubSystem Specifications/Application Functions - EA4/SF033A Vehicle Signal Conditioning)' '#SF033A_97' 'true' 'REQ:  SF033A_97' '' } %GIDa_2f71fb1f_a485_4d70_97a9_5400811bedd1"  Port=2  PortDimensions=1
  Action Port : ActionPort  ActionType=then
  Constant : Constant  RequirementInfo="{'linktype_rmi_doors' '00012fc2 (/E-STEER Core/SubSystem Specifications/Application Functions - EA4/SF033A Vehicle Signal Conditioning)' '#SF033A_97' 'true' 'REQ:  SF033A_97' '' } %GIDa_11d24f3d_4250_4669_bae2_03ee3ec4b2fd"  Value=KPHCONVTOMTRPERSEC_MTRPERSECPERKPH_F32
  Constant1 : Constant  RequirementInfo="{'linktype_rmi_doors' '00012fc2 (/E-STEER Core/SubSystem Specifications/Application Functions - EA4/SF033A Vehicle Signal Conditioning)' '#SF033A_97' 'true' 'REQ:  SF033A_97' '' } %GIDa_02e9ee95_81fa_44c3_aae7_fac6799d10c7"  Value=ARCHGLBPRM_180OVERPI_ULS_F32
  Divide : Product  RequirementInfo="{'linktype_rmi_doors' '00012fc2 (/E-STEER Core/SubSystem Specifications/Application Functions - EA4/SF033A Vehicle Signal Conditioning)' '#SF033A_97' 'true' 'REQ:  SF033A_97' '' } %GIDa_2baea36b_825c_40b7_9c93_9c8590ccc077"  Inputs=*/
  Product : Product  RequirementInfo="{'linktype_rmi_doors' '00012fc2 (/E-STEER Core/SubSystem Specifications/Application Functions - EA4/SF033A Vehicle Signal Conditioning)' '#SF033A_97' 'true' 'REQ:  SF033A_97' '' } %GIDa_78220a1b_26e4_4745_84e0_7bc9616064c6"
  Product1 : Product  RequirementInfo="{'linktype_rmi_doors' '00012fc2 (/E-STEER Core/SubSystem Specifications/Application Functions - EA4/SF033A Vehicle Signal Conditioning)' '#SF033A_97' 'true' 'REQ:  SF033A_97' '' } %GIDa_395bf554_61c1_4b65_9a16_a8c4cab846e5"
  VehLatAEstimd : Outport  RequirementInfo="{'linktype_rmi_doors' '00012fc2 (/E-STEER Core/SubSystem Specifications/Application Functions - EA4/SF033A Vehicle Signal Conditioning)' '#SF033A_97' 'true' 'REQ:  SF033A_97' '' } %GIDa_839fea7b_f146_4653_b9b2_3c9a04c97a12"
  wires:
  Constant1/1 -> Product/2
  VehYawRate/1 -> Product/1
  Constant/1 -> Divide/2
  VehSpd/1 -> Divide/1
  Product/1 -> Product1/1
  Divide/1 -> Product1/2
  Product1/1 -> VehLatAEstimd/1

== system SF033A_VehSigCdng/VehSigCdng/VehSigCdngPer1/Lateral Acceleration Estimation/CopyRight2 ==

== system SF033A_VehSigCdng/VehSigCdng/VehSigCdngPer1/Lateral Acceleration Estimation/SetDefaultValue ==
  Action Port : ActionPort  ActionType=else
  Constant10 : Constant  RequirementInfo="{'linktype_rmi_doors' '00012fc2 (/E-STEER Core/SubSystem Specifications/Application Functions - EA4/SF033A Vehicle Signal Conditioning)' '#SF033A_99' 'true' 'REQ:  SF033A_99' '' } %GIDa_c98059b6_d376_4216_b1c0_9c812a7f1bad"  Value=VehSigCdngDftLatA
  DefaultValue : Outport  RequirementInfo="{'linktype_rmi_doors' '00012fc2 (/E-STEER Core/SubSystem Specifications/Application Functions - EA4/SF033A Vehicle Signal Conditioning)' '#SF033A_99' 'true' 'REQ:  SF033A_99' '' } %GIDa_21c5de6d_6dbf_4072_adf1_58d1c8b2a15f"
  wires:
  Constant10/1 -> DefaultValue/1

== system SF033A_VehSigCdng/VehSigCdng/VehSigCdngPer1/Longitudinal Acceleration/CopyRight2 ==

== system SF033A_VehSigCdng/VehSigCdng/VehSigCdngPer1/Longitudinal Acceleration/FltInj_Sim ==
  note: This block requires no modification by FDD author.
      |
      | This block does not actually simulate any fault injection.  It is simply a pass-thru.
      |
      | The Enum port (#2) simply terminates its signal, but we are trying to force the FDD author
      | to properly use the FltInjectionLocType enumeration in FDD model.
  note: EA4.x Fault Injection
  note: Inport #2 must be enumeration
      | Enum: FltInjectionLocType
  Signal : Inport
  Enum : Inport  Port=2
  Terminator : Terminator
  Out1 : Outport
  wires:
  Signal/1 -> Out1/1
  Enum/1 -> Terminator/1

== system SF033A_VehSigCdng/VehSigCdng/VehSigCdngPer1/Longitudinal Acceleration/If_NotVld ==
  In1 : Inport
  Action Port : ActionPort  ActionType=else
  CopyRight2 : Subsystem  Description=|  mask(Copyright Information){none=on}
      | Copyright info block.                                               
      |                                                                     
      | Place copyright information at the top of every subsystem in design.
      mask prompts: none "No parameters"
      mask help: Place copyright information at the top of every subsystem in design.
      mask Display:
      | NxtrConf = 'Nexteer Confidential';
      | 
      | sys = bdroot; %handle for the current model ("system")
      | first = get_param(sys,'Created');
      | first = first(end-3:end);  %year is last four digits
      | 
      | last = get_param(sys,'LastModifiedDate');
      | if isempty(last)
      |     last = datestr(now,'yyyy');
      | else
      |     last = last(end-3:end);
      | end
      | 
      | if strcmp(first,last)
      |     fprintf('%s -- Copyright %s Nexteer',NxtrConf,first)
      | else
      |     fprintf('%s -- %s%s- %s Nexteer',NxtrConf,char(169),first,last)
      | end
  Out1 : Outport
  wires:
  In1/1 -> Out1/1

== system SF033A_VehSigCdng/VehSigCdng/VehSigCdngPer1/Longitudinal Acceleration/If_Vld ==
  In1 : Inport
  Action Port : ActionPort  ActionType=then
  CopyRight2 : Subsystem  Description=|  mask(Copyright Information){none=on}
      | Copyright info block.                                               
      |                                                                     
      | Place copyright information at the top of every subsystem in design.
      mask prompts: none "No parameters"
      mask help: Place copyright information at the top of every subsystem in design.
      mask Display:
      | NxtrConf = 'Nexteer Confidential';
      | 
      | sys = bdroot; %handle for the current model ("system")
      | first = get_param(sys,'Created');
      | first = first(end-3:end);  %year is last four digits
      | 
      | last = get_param(sys,'LastModifiedDate');
      | if isempty(last)
      |     last = datestr(now,'yyyy');
      | else
      |     last = last(end-3:end);
      | end
      | 
      | if strcmp(first,last)
      |     fprintf('%s -- Copyright %s Nexteer',NxtrConf,first)
      | else
      |     fprintf('%s -- %s%s- %s Nexteer',NxtrConf,char(169),first,last)
      | end
  Out1 : Outport
  wires:
  In1/1 -> Out1/1

== system SF033A_VehSigCdng/VehSigCdng/VehSigCdngPer1/Vehicle Speed/CopyRight2 ==

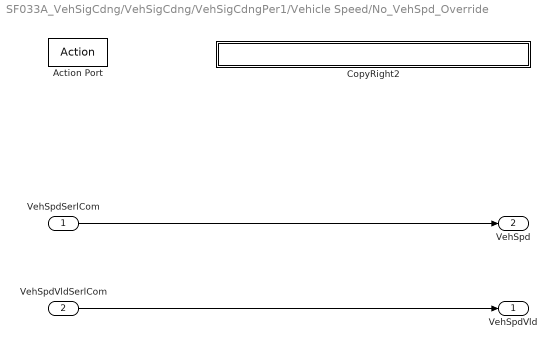
== system SF033A_VehSigCdng/VehSigCdng/VehSigCdngPer1/Vehicle Speed/No_VehSpd_Override ==
  VehSpdSerlCom : Inport  PortDimensions=1
  VehSpdVldSerlCom : Inport  Port=2  PortDimensions=1
  Action Port : ActionPort  ActionType=else
  CopyRight2 : Subsystem  Description=|  mask(Copyright Information){none=on}
      | Copyright info block.                                               
      |                                                                     
      | Place copyright information at the top of every subsystem in design.
      mask prompts: none "No parameters"
      mask help: Place copyright information at the top of every subsystem in design.
      mask Display:
      | NxtrConf = 'Nexteer Confidential';
      | 
      | sys = bdroot; %handle for the current model ("system")
      | first = get_param(sys,'Created');
      | first = first(end-3:end);  %year is last four digits
      | 
      | last = get_param(sys,'LastModifiedDate');
      | if isempty(last)
      |     last = datestr(now,'yyyy');
      | else
      |     last = last(end-3:end);
      | end
      | 
      | if strcmp(first,last)
      |     fprintf('%s -- Copyright %s Nexteer',NxtrConf,first)
      | else
      |     fprintf('%s -- %s%s- %s Nexteer',NxtrConf,char(169),first,last)
      | end
  VehSpdVld : Outport
  VehSpd : Outport  Port=2
  wires:
  VehSpdSerlCom/1 -> VehSpd/1
  VehSpdVldSerlCom/1 -> VehSpdVld/1

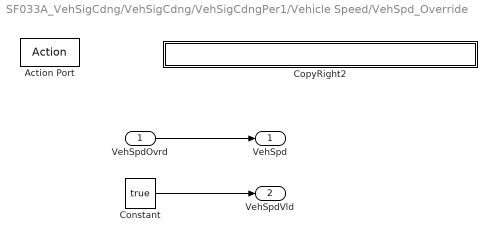
== system SF033A_VehSigCdng/VehSigCdng/VehSigCdngPer1/Vehicle Speed/VehSpd_Override ==
  VehSpdOvrd : Inport  RequirementInfo="{'linktype_rmi_doors' '00012fc2 (/E-STEER Core/SubSystem Specifications/Application Functions - EA4/SF033A Vehicle Signal Conditioning)' '#SF033A_70' 'true' 'REQ:  SF033A_70' '' ; 'linktype_rmi_doors' '00012fc2 (/E-STEER Core/SubSystem Specifications/Application Functions - EA4/SF033A Vehicle Signal Conditioning)' '#SF033A_106' 'true' 'REQ:  SF033A_106' '' } %GIDa_1bc77041_e7ca_41b3_a18e_4ebf3953f159"
  Action Port : ActionPort  ActionType=then
  Constant : Constant  RequirementInfo="{'linktype_rmi_doors' '00012fc2 (/E-STEER Core/SubSystem Specifications/Application Functions - EA4/SF033A Vehicle Signal Conditioning)' '#SF033A_70' 'true' 'REQ:  SF033A_70' '' ; 'linktype_rmi_doors' '00012fc2 (/E-STEER Core/SubSystem Specifications/Application Functions - EA4/SF033A Vehicle Signal Conditioning)' '#SF033A_106' 'true' 'REQ:  SF033A_106' '' } %GIDa_230667f1_616e_4319_a899_0076bcdd9aff"  Value=true  OutDataTypeStr=boolean
  CopyRight2 : Subsystem  Description=|  mask(Copyright Information){none=on}
      | Copyright info block.                                               
      |                                                                     
      | Place copyright information at the top of every subsystem in design.
      mask prompts: none "No parameters"
      mask help: Place copyright information at the top of every subsystem in design.
      mask Display:
      | NxtrConf = 'Nexteer Confidential';
      | 
      | sys = bdroot; %handle for the current model ("system")
      | first = get_param(sys,'Created');
      | first = first(end-3:end);  %year is last four digits
      | 
      | last = get_param(sys,'LastModifiedDate');
      | if isempty(last)
      |     last = datestr(now,'yyyy');
      | else
      |     last = last(end-3:end);
      | end
      | 
      | if strcmp(first,last)
      |     fprintf('%s -- Copyright %s Nexteer',NxtrConf,first)
      | else
      |     fprintf('%s -- %s%s- %s Nexteer',NxtrConf,char(169),first,last)
      | end
  VehSpd : Outport  RequirementInfo="{'linktype_rmi_doors' '00012fc2 (/E-STEER Core/SubSystem Specifications/Application Functions - EA4/SF033A Vehicle Signal Conditioning)' '#SF033A_70' 'true' 'REQ:  SF033A_70' '' ; 'linktype_rmi_doors' '00012fc2 (/E-STEER Core/SubSystem Specifications/Application Functions - EA4/SF033A Vehicle Signal Conditioning)' '#SF033A_106' 'true' 'REQ:  SF033A_106' '' } %GIDa_672694d9_7d30_46e5_952d_32f1a1905b64"
  VehSpdVld : Outport  RequirementInfo="{'linktype_rmi_doors' '00012fc2 (/E-STEER Core/SubSystem Specifications/Application Functions - EA4/SF033A Vehicle Signal Conditioning)' '#SF033A_70' 'true' 'REQ:  SF033A_70' '' ; 'linktype_rmi_doors' '00012fc2 (/E-STEER Core/SubSystem Specifications/Application Functions - EA4/SF033A Vehicle Signal Conditioning)' '#SF033A_106' 'true' 'REQ:  SF033A_106' '' } %GIDa_b5cfd0fb_ef99_4707_81ad_c77a2296a526"  Port=2
  wires:
  VehSpdOvrd/1 -> VehSpd/1
  Constant/1 -> VehSpdVld/1
